simulink model "observermodel"  (R2020a)
settings: Solver=VariableStepAuto  StartTime=0.0  StopTime=U1(end,1)  RelTol=1e-3
values from neighbouring files (symbols this model uses):
  C = C    [Observer_mat.m]    (also in discretemodel.mat = [0  0  1  0; 0  0  0  1]; lqr_whitebox.m = sys.C; lqr_whitebox.mat = [0  0  1  0; 0  0  0  1]; matrices.mat = [0  0  1  0; 0  0  0  1])
  gamma = B    [Observer_mat.m]    (also in discretemodel.mat = [0.004353030085  4.48398112985e-06; 6.47055504813e-06  0.003; observer_matlab.m = Ad.B; observermatlab.m = Ad.B)
  h = tout(2)-tout(1)    [Linearize_whitebox.m]    (also in Linearize_whitebox_final.m; Observer_mat.m; lqr_whitebox.mat = 1.00037043897; matrices.mat = 1.00080032013)
  K = [0.871464143609  0.0262786205748; 0.0262786205748  0.871464143609; 0.341518856741  0.00295216925623; 0.00295216925623  0.341518856741]    [K_matrix.mat]    (also in K_matrix_final.mat = [0.107540648809  0.00297468629139; 0.00297468629139  0.10754; Observer_mat.m = place(phi.',C.',P).'; lqr_whitebox.m = lqr(A,B,Q,R); lqr_whitebox.mat = [9.8403850338  0.823629600444  7.09136571585  0.104667034235)
  phi = A    [Observer_mat.m]    (also in discretemodel.mat = [0.991639753181 0.00295216925623 0.0399517774449 5.979211225; observer_matlab.m = Ad.A; observermatlab.m = Ad.A)
undefined symbols (not defined in the file or in its folder): DiscIntNeverNeededParam
settings Model: Creator=SIDTUDelft1  LastModifiedBy=Eveline
settings DataIOCC: ReturnWorkspaceOutputs=off

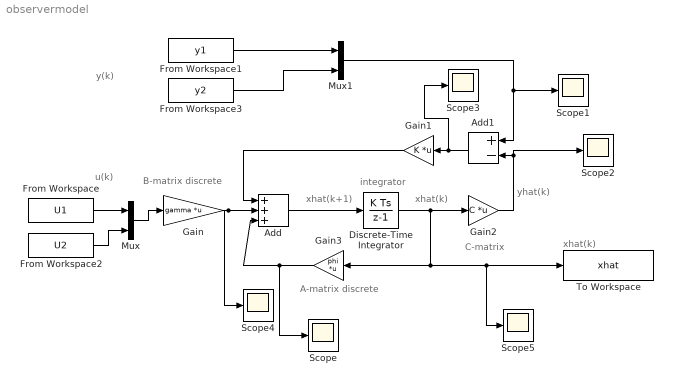
== system observermodel ==
  note: C-matrix
  note: integrator
  note: A-matrix discrete
  note: B-matrix discrete
  note: xhat(k)
  note: yhat(k)
  note: xhat(k)
  note: xhat(k+1)
  note: u(k)
  note: y(k)
  Add : Sum  Inputs=+++
  Add1 : Sum  Inputs=+-
  Discrete-Time Integrator : DiscreteIntegrator  InitialCondition=300  SampleTime=-1  ICPrevOutput=DiscIntNeverNeededParam  ICPrevScaledInput=DiscIntNeverNeededParam
  From Workspace : FromWorkspace  VariableName=U1  SampleTime=h
  From Workspace1 : FromWorkspace  VariableName=y1  SampleTime=h
  From Workspace2 : FromWorkspace  VariableName=U2  SampleTime=h
  From Workspace3 : FromWorkspace  VariableName=y2  SampleTime=h
  Gain : Gain  Gain=gamma  Multiplication=Matrix(K*u)
  Gain1 : Gain  Gain=K  Multiplication=Matrix(K*u)
  Gain2 : Gain  Gain=C  Multiplication=Matrix(K*u)
  Gain3 : Gain  Gain=phi  Multiplication=Matrix(K*u)
  Mux : Mux  Inputs=2
  Mux1 : Mux  Inputs=2
  Scope{,1..5} (6 alike) : Scope
  To Workspace : ToWorkspace  VariableName=xhat  SampleTime=h
  wires:
  Gain/1 -> Scope4/1, Add/2
  From Workspace1/1 -> Mux1/1
  Add1/1 -> Scope3/1, Gain1/1
  Gain1/1 -> Add/1
  Add/1 -> Discrete-Time Integrator/1
  Discrete-Time Integrator/1 -> Scope5/1, To Workspace/1, Gain3/1, Gain2/1
  Gain2/1 -> Scope2/1, Add1/2
  Gain3/1 -> Scope/1, Add/3
  From Workspace/1 -> Mux/1
  From Workspace2/1 -> Mux/2
  Mux/1 -> Gain/1
  From Workspace3/1 -> Mux1/2
  Mux1/1 -> Scope1/1, Add1/1
